simulink model "lungModel1"  (R2022a)
settings: Solver=FixedStepAuto  StartTime=0.0  StopTime=470.0  FixedStep=0.05  RelTol=1e-3
model workspace (MAT data in the model file):
  B = 760
  Mdot = 3.8
  Mu_c = -1445
  Mu_p = -1250
  P1 = 0.3
  V_T = 500
  Vt = 15000
  alpha = 0.0065
  alpha1 = 0.8
  lambda_c = 33.3
  lambda_p = 33.3
  qdot = 100
libraries: fod x2
settings Model: Creator=mrmog  LastModifiedBy=mrmog
settings DebuggingCC: UnderSpecifiedDimensionMsg=warning

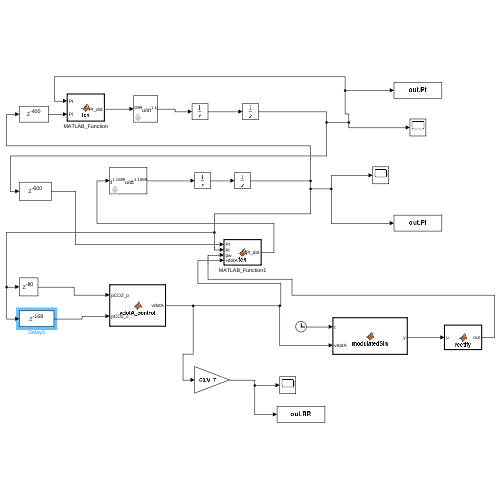
[thumbnail: Simulink's stored preview of the top-level diagram]
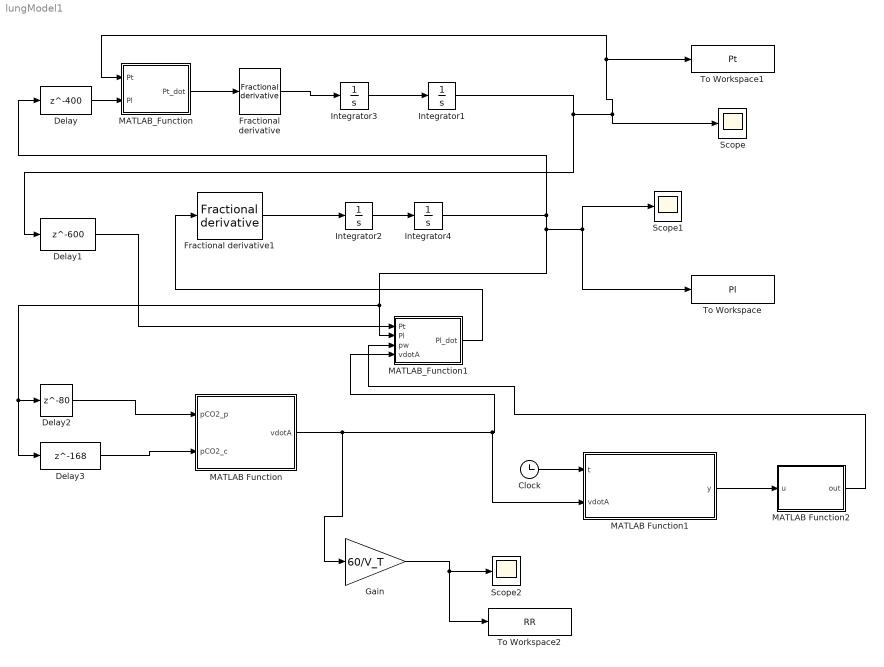
== system lungModel1 ==
  Clock : Clock
  Delay : Delay  DelayLength=400  InitialCondition=41.6
  Delay1 : Delay  DelayLength=600  InitialCondition=47.3
  Delay2 : Delay  DelayLength=80  InitialCondition=41.6
  Delay3 : Delay  DelayLength=168  InitialCondition=41.6
  Fractional derivative : fod/Fractional derivative  gam=alpha1  ww=[0.001; 20]  n=20  nFod=off
      settings: SourceProductName=FOMCON Toolbox
  Fractional derivative1 : fod/Fractional derivative  gam=alpha1  ww=[0.001; 20]  n=20  nFod=off
      settings: SourceProductName=FOMCON Toolbox
  Gain : Gain  Gain=60/V_T
  Integrator1 : Integrator  InitialCondition=47.6
  Integrator2 : Integrator
  Integrator3 : Integrator
  Integrator4 : Integrator  InitialCondition=41.3
  MATLAB Function : MATLAB Function  TreatAsAtomicUnit=on
  MATLAB Function1 : MATLAB Function  TreatAsAtomicUnit=on
  MATLAB Function2 : MATLAB Function  TreatAsAtomicUnit=on
  MATLAB_Function : MATLAB Function  TreatAsAtomicUnit=on
  MATLAB_Function1 : MATLAB Function  TreatAsAtomicUnit=on
  Scope : Scope
  Scope1 : Scope
  Scope2 : Scope
  To Workspace : ToWorkspace  VariableName=Pl  SaveFormat=Timeseries  SampleTime=-1
  To Workspace1 : ToWorkspace  VariableName=Pt  SaveFormat=Timeseries  SampleTime=-1
  To Workspace2 : ToWorkspace  VariableName=RR  SaveFormat=Timeseries  SampleTime=-1
  wires:
  Delay/1 -> MATLAB_Function/2(Pl)
  Delay1/1 -> MATLAB_Function1/1(Pt)
  MATLAB Function/1(vdotA) -> Gain/1, MATLAB Function1/2(vdotA), MATLAB_Function1/4(vdotA)
  Delay2/1 -> MATLAB Function/1(pCO2_p)
  Delay3/1 -> MATLAB Function/2(pCO2_c)
  Clock/1 -> MATLAB Function1/1(t)
  MATLAB Function1/1(y) -> MATLAB Function2/1(u)
  MATLAB Function2/1(out) -> MATLAB_Function1/3(pw)
  Gain/1 -> To Workspace2/1, Scope2/1
  Integrator4/1 -> MATLAB_Function1/2(Pl), Delay3/1, Delay2/1, To Workspace/1, Scope1/1, Delay/1
  Integrator1/1 -> Delay1/1, Scope/1, MATLAB_Function/1(Pt), To Workspace1/1
  MATLAB_Function1/1(Pl_dot) -> Fractional derivative1/1
  MATLAB_Function/1(Pt_dot) -> Fractional derivative/1
  Integrator2/1 -> Integrator4/1
  Integrator3/1 -> Integrator1/1
  Fractional derivative/1 -> Integrator3/1
  Fractional derivative1/1 -> Integrator2/1

== matlab function lungModel1/MATLAB_Function1 ==
  data: Pt input; Pl input; pw input; Pl_dot output; vdotA input
function Pl_dot = fcn(Pt,Pl,pw,vdotA)

Fp=100;

B = 760;

P1 = 0.3;

%V_T=500;
Vl=3200;

alpha = 0.0065;

%Pl_dot = ((lambda_c*P1 + alpha*qdot*B)/Vl)*Pt - ((alpha*qdot*B + Mu_c+ vldot/B)/Vl)*Pl - (lambda_c/Vl)*Pt*Pl + Mu_c*P1/Vl;
%Pl_dot = (alpha*Fp*B/Vl)*Pt - ((alpha*Fp*B + (1-pulsewav1(t,V_T/vdotA))*vdotA)/Vl)*Pl + (pusewav1(t,V_T/vdotA)*vdotA*P1)/Vl;
Pl_dot = (alpha*Fp*B/Vl)*Pt - ((alpha*Fp*B + (1-pw)*vdotA)/Vl)*Pl + (pw*vdotA*P1)/Vl;

== matlab function lungModel1/MATLAB_Function ==
  data: Pt input; Pt_dot output; Pl input
function Pt_dot = fcn(Pt,Pl)

qdot = 100;
Mdot = 3.8;
Vt = 15000;
alpha = 0.0065;

Pt_dot = (-qdot/Vt)*Pt + (qdot/Vt)*Pl + (Mdot/(alpha*Vt));

== matlab function lungModel1/MATLAB Function ==
  data: pCO2_p input; vdotA output; pCO2_c input
function vdotA = vdotA_control(pCO2_p,pCO2_c)

%GP=500*exp(-0.05*82);
%GP=387.5*exp(-0.05*99);
GP=2000*exp(-0.05*82);
IP=39;
%IP=33;
MRB=50/60;
%MRB=11/60;
KCO2=0.0057;
%KCO2=0.005;
FB=80;
%FB=238/60;
IC=39;
%IC=33;
GC=1500/60;
%GC=22.8;

Mu_c = -GC*(MRB/(KCO2*FB) + IC);
%Mu_c = Mu_c;
Mu_p=-GP*IP;
lambda_c=GC;
lambda_p=GP;

vdotA = max(0,lambda_c*pCO2_c + Mu_c)+max(0,lambda_p*pCO2_p + Mu_p);

== matlab function lungModel1/MATLAB Function1 ==
  data: t input; y output; vdotA input
function y = modulatedSin(t,vdotA)

V_T = 500;
f = vdotA/V_T;

y = sin(2*pi*f*t);

== matlab function lungModel1/MATLAB Function2 ==
  data: u input; out output
function out = rectify(u)

if u>0
    out=1;
else
    out=0;
end
